simulink model "ssc_lithium_cell_1RC_testPulseData"  (R2022b)
settings: Solver=ode15s  StartTime=0.0  StopTime=40000  MaxStep=60  RelTol=1e-3  EnableMultiTasking=on
PreLoadFcn:
  | ssc_lithium_cell_1RC_ini
undefined symbols (not defined in the file or in its folder): sigbuilder_block
libraries: fl_lib x6, nesl_utility x4, LiBatteryBlocks x1
Description:
  | Lithium Battery Cell - One RC-Branch Equivalent Circuit
  | 
  | This example shows how to model a lithium cell using the Simscape(TM)
  | language to implement the elements of an equivalent circuit model
  | with one RC branch. For the defining equations and their validation,
  | see T. Huria, M. Ceraolo, J. Gazzarri, R. Jackey. "High Fidelity Electrical
  | Model with Thermal Dependence for Characterization and Simulation of
  | High Power Lithium Battery Cells," IEEE International Electric Vehicle
  | Conference, March 2012.
  | 
  | A simple thermal model is used to model battery temperature. It is
  | assumed that cooling is primarily via convection, and that heating is
  | primarily from internal resistance. A battery pack can be modeled by
  | connecting multiple copies of the battery cell block in series.
  | 
  | 
  | 
  | Copyright 2008-2012 The MathWorks, Inc.
settings Model: Creator=MathWorks  LastModifiedBy=Loki
settings SolverCC: AlgebraicLoopSolver=TrustRegion
settings DataIOCC: ExternalInput=[PulseData.time, PulseData.current, PulseData.temperature]  LimitDataPoints=on  LoadExternalInput=on  SaveFormat=Array  SignalLoggingSaveFormat=ModelDataLogs  ReturnWorkspaceOutputs=off
settings OptimizationCC: ExpressionDepthLimit=2147483647  LifeSpan=inf
settings DebuggingCC: UnderspecifiedInitializationDetection=Classic  MergeDetectMultiDrivingBlocksExec=none  FcnCallInpInsideContextMsg=warning  UnconnectedInputMsg=warning  UnconnectedOutputMsg=warning  UnconnectedLineMsg=warning  StateNameClashWarn=warning  SFUnexpectedBacktrackingDiag=warning  SFNoUnconditionalDefaultTransitionDiag=warning  SFExecutionAtInitializationDiag=none  SFMachineParentedDataDiag=warning  ArithmeticOperatorsInVariantConditions=warning
settings HardwareCC: ProdBitPerPointer=32  ProdBitPerSizeT=32  ProdBitPerPtrDiffT=32  ProdLargestAtomicFloat=None  ProdIntDivRoundTo=Undefined  ProdEndianess=Unspecified  ProdWordSize=32  ProdHWDeviceType=32-bit Generic
settings ModelReferenceCC: EnableRefExpFcnMdlSchedulingChecks=on  PropagateSignalLabelsOutOfModel=off
settings SFSimCC: SimUseLocalCustomCode=off  CustomCodeUndefinedFunction=UseInterfaceOnly
settings RTWCC: RTWUseLocalCustomCode=off
settings CodeAppCC: StateflowObjectComments=on
settings GRTTargetCC: TargetLangStandard=C89/C90 (ANSI)  CombineOutputUpdateFcns=off  GRTInterface=on
settings ConfigComp: CovMetricSettings=dw  CovSaveCumulativeToWorkspaceVar=on  CovSaveSingleToWorkspaceVar=on  CovExternalEMLEnable=off
settings SimscapeCC: SimscapeNormalizeSystem=off

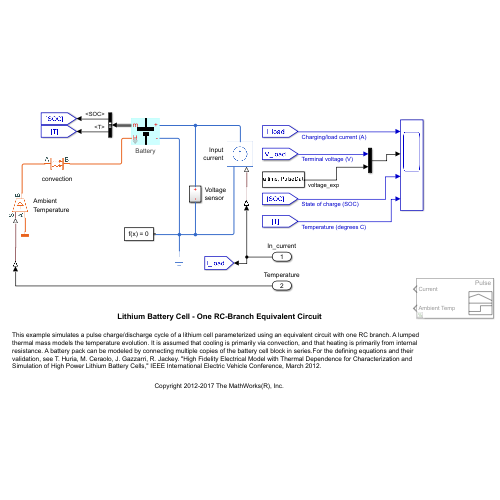
[thumbnail: Simulink's stored preview of the top-level diagram]
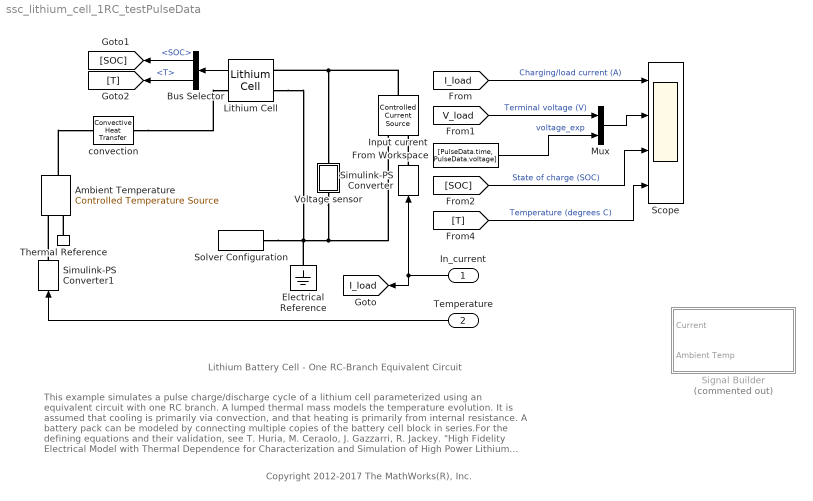
== system ssc_lithium_cell_1RC_testPulseData ==
  note: Lithium Battery Cell - One RC-Branch Equivalent Circuit
  note: This example simulates a pulse charge/discharge cycle of a lithium cell parameterized using an equivalent circuit with one RC branch. A lumped thermal mass models the temperature evolution. It is assumed that cooling is primarily via convection, and that heating is primarily from internal resistance. A battery pack can be modeled by connecting multiple copies of the battery cell block in series.For the defining equations and their validation, see T. Huria, M. Ceraolo, J. Gazzarri, R. Jackey. "High Fidelity Electrical Model with Thermal Dependence for Characterization and Simulation of High Power Lithium Battery Cells," IEEE International Electric Vehicle Conference, March 2012.
  note: Copyright 2012-2017 The MathWorks(R), Inc.
  In_current : Inport
  Temperature : Inport  Port=2
  Ambient Temperature : fl_lib/Thermal/Thermal Sources/Controlled Temperature Source
  Bus Selector : BusSelector  OutputSignals=SOC,T
  Electrical Reference : fl_lib/Electrical/Electrical Elements/Electrical Reference
  From Workspace : FromWorkspace  VariableName=[PulseData.time, PulseData.voltage]
  Input current : fl_lib/Electrical/Electrical Sources/Controlled Current Source
  Lithium Cell : LiBatteryBlocks/Lithium Cell  Battery=Battery
      settings: AttributesFormatString=%<Battery>
  Mux : Mux  Inputs=2
  Scope : Scope  NumInputPorts=4
  Signal Builder : Subsystem  Tag=STV Subsys  Commented=on  LoadFcn=sigbuilder_block('load');  StartFcn=sigbuilder_block('start');  StopFcn=sigbuilder_block('stop');  ClipboardFcn=sigbuilder_block('clipboard');  mask(Sigbuilder block){tuvar=[0:10]}
      mask help: Simulink:masks:SigbuilderBlock_MD
      mask init:
      | if ~strcmp(get_param(bdroot(gcbh),'SimulationStatus'),'stopped') tuvar = sigbuilder_block('maskInit'); end
      settings: CopyFcn=sigbuilder_block('copy');  DeleteFcn=sigbuilder_block('delete');  ModelCloseFcn=sigbuilder_block('modelClose');  PreSaveFcn=sigbuilder_block('preSave');  PauseFcn=sigbuilder_block('pause');  ContinueFcn=sigbuilder_block('continue');  NameChangeFcn=sigbuilder_block('namechange');  OpenFcn=sigbuilder_block('open',[33.75 101.25 755.25 399.75 ]);  CloseFcn=sigbuilder_block('close');
      mask Display: plot(0, 0, 100, 100,[2, 2, 32, 32, 2], [68, 8, 8, 68, 68],[32, 2], [38, 38], [32, 19, 2],[53, 60, 44], [32, 17, 17, 2],[16, 16, 31, 31]);txt = getActiveGroup(gcbh);text(2, 100, txt,'verticalAlignment', 'top');
  Simulink-PS Converter : nesl_utility/Simulink-PS Converter  PhysicalDomain=network_engine_domain  SubClassName=ps_input  LeftPortType=input  RightPortType=output  PseudoPeriodic=off  Frequencies=[]  NoiseDistribution=none  NoiseParameters=[]  Unit=A  AffineConversion=off  FilteringAndDerivatives=zero  SimscapeFilterOrder=1  InputFilterTimeConstant=.001  UdotUserProvided=1
  Simulink-PS Converter1 : nesl_utility/Simulink-PS Converter  PhysicalDomain=network_engine_domain  SubClassName=ps_input  LeftPortType=input  RightPortType=output  PseudoPeriodic=off  Frequencies=[]  NoiseDistribution=none  NoiseParameters=[]  Unit=degC  AffineConversion=on  FilteringAndDerivatives=zero  SimscapeFilterOrder=1  InputFilterTimeConstant=.001  UdotUserProvided=1
  Solver Configuration : nesl_utility/Solver Configuration  PhysicalDomain=network_engine_domain  SubClassName=solver  LeftPortType=input  RightPortType=generic  Tones=[]  Harmonics=[]  SimulateNoise=off  Profile=off  UseLocalSampling=off  EnableSwitchedLinearOptims=on  FrequencyDomain=off  UseCCode=off  RelTol=0.001  AbsTol=1e-06  MinStep=1e-09  ToWorkspace=off  RevertToSquareIcSolve=off  NumHomotopyIterations=100  PhasorMode=off  PhasorModeNumHarmonics=1  ConsistencySolver=NEWTON_FTOL  IndexReductionMethod=DerivativeReplacement  DoDC=off  ResidualTolerance=1e-9  ConsistencyTolSource=GLOBAL  ConsistencyAbsTol=0.001  ConsistencyRelTol=0.001  ConsistencyTolFactor=0.001  UseLocalSolver=off  LocalSolverChoice=NE_BACKWARD_EULER_ADVANCER  ResolveIndetEquations=on  FunctionEvalNumThread=1  LocalSolverSampleTime=1  DoFixedCost=off  MaxNonlinIter=3  MaxModeIter=2  ComputeImpulses=off  ImpulseIterations=2  LinearAlgebra=Sparse  LinearAlgebraNumThread=0  EquationFormulation=NE_TIME_EF  DelaysMemoryBudget=1024  AutomaticFiltering=on  FilteringTimeConstant=0.001  PartitionStorageMethod=AS_NEEDED  PartitionMemoryBudget=1024  PartitionMethod=FAST
  Thermal Reference : fl_lib/Thermal/Thermal Elements/Thermal Reference
  Voltage sensor : Subsystem
  convection : fl_lib/Thermal/Thermal Elements/Convective Heat Transfer  thermal_type=foundation.enum.constant_variable.constant  area=cell_area m^2  heat_tr_coeff=h_conv W/(m^2 * K)  min_heat_tr_coeff=1e-3 W/(K*m^2)  T_specify=off  T_priority=None  T=0 K  T_nominal_specify=off  T_nominal_unit=K  T_nominal_value=1  Q_specify=off  Q_priority=None  Q=0 J/s  Q_nominal_specify=off  Q_nominal_unit=J/s  Q_nominal_value=1
  tag scope: I_load=global
  wires:
  [SOC] -> Scope/3  "State of charge (SOC)"
  [T] -> Scope/4  "Temperature (degrees C)"
  [I_load] -> Scope/1  "Charging/load current (A)"
  In_current/1 -> [I_load], Simulink-PS Converter/1
  Lithium Cell/1 -> Bus Selector/1
  Bus Selector/1 -> [SOC]  "<SOC>"
  Bus Selector/2 -> [T]  "<T>"
  [V_load] -> Mux/1  "Terminal voltage (V)"
  Mux/1 -> Scope/2
  From Workspace/1 -> Mux/2  "voltage_exp"
  Temperature/1 -> Simulink-PS Converter1/1
  connections:
  Electrical Reference/LConn1 -- Input current/RConn2 -- Voltage sensor/RConn1 -- Lithium Cell/LConn2 -- Solver Configuration/RConn1
  Input current/LConn1 -- Lithium Cell/LConn1 -- Voltage sensor/LConn1
  Thermal Reference/LConn1 -- Ambient Temperature/RConn2
  Ambient Temperature/LConn1 -- convection/LConn1
  convection/RConn1 -- Lithium Cell/RConn1
  Simulink-PS Converter/RConn1 -- Input current/RConn1
  Simulink-PS Converter1/RConn1 -- Ambient Temperature/RConn1

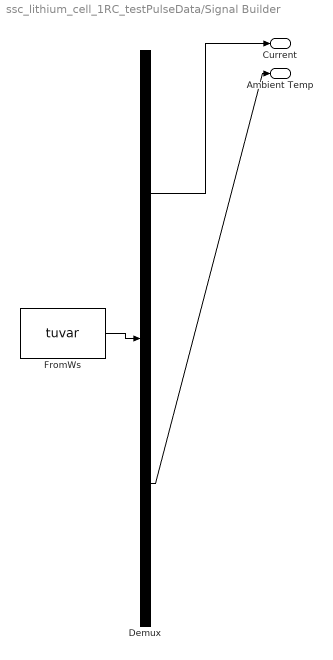
== system ssc_lithium_cell_1RC_testPulseData/Signal Builder ==
  Demux : Demux  Tag=STV Demux  Outputs=2
      settings: DisplayOption=none
  FromWs : FromWorkspace  Tag=STV FromWs  VariableName=tuvar
      SigBuilderData=|
      | common.afterFinalStr = 'Extrapolate'
      | common.sampleTime = 0
      | dataSet(1).timeRange = [0 40000]
      | dataSet(1).name = 'Pulse'
      | dataSet(2).timeRange = [0 40000]
      | dataSet(2).name = 'Constant'
      | sbobj.Name = 'Signal Builder'
      | sbobj.Groups(1).Name = 'Pulse'
      | sbobj.Groups(1).Signals(1).Name = 'Current'
      | sbobj.Groups(1).Signals(1).XData = [0 300 300 2100 2100 3600 3600 3960 3960 7200 7200 7560 7560 10800 10800 11160 11160 14400 14400 14760 14760 18000 18000 18360 18360 21600 21600 21960 21960 25200 25200 25560 25560 28800 28800 29160 29160 32400 32400 32760 32760 36000 36000 36360 36360 40000]
      | sbobj.Groups(1).Signals(1).YData = [0 0 31.5 31.5 0 0 -27.625 -27.625 0 0 -27.625 -27.625 0 0 -27.625 -27.625 0 0 -27.625 -27.625 0 0 -27.625 -27.625 0 0 -27.625 -27.625 0 0 -27.625 -27.625 0 0 -27.625 -27.625 0 0 -27.625 -27.625 0 0 -27.625 -27.625 0 0]
      | sbobj.Groups(1).Signals(2).Name = 'Ambient Temp'
      | sbobj.Groups(1).Signals(2).XData = [0 300 2100 3600 3960 7200 7560 10800 11160 14400 14760 18000 18360 21600 21960 25200 25560 28800 29160 32400 32760 36000 36360 40000]
      | sbobj.Groups(1).Signals(2).YData = [20 20 20 20 20 20 20 20 20 20 20 20 20 20 20 20 20 20 20 20 20 20 20 20]
      | sbobj.Groups(1).TimeRange = [0 40000]
      | sbobj.Groups(2).Name = 'Constant'
      | sbobj.Groups(2).Signals(1).Name = 'Current'
      | sbobj.Groups(2).Signals(1).XData = [0 360 360 9100 9100 11800 11800 28200 33800 40000]
      | sbobj.Groups(2).Signals(1).YData = [0 0 -5 -5 0 0 5 5 0 0]
      | sbobj.Groups(2).Signals(2).Name = 'Ambient Temp'
      | sbobj.Groups(2).Signals(2).XData = [0 360 360 9100 9100 11800 11800 28200 33800 40000]
      | sbobj.Groups(2).Signals(2).YData = [20 20.09 20.09 22.275 22.275 22.95 22.95 27.05 28.45 30]
      | sbobj.Groups(2).TimeRange = [0 40000]
  Current : Outport
  Ambient Temp : Outport  Tag=STV Outport  Port=2
  wires:
  Demux/1 -> Current/1
  FromWs/1 -> Demux/1
  Demux/2 -> Ambient Temp/1

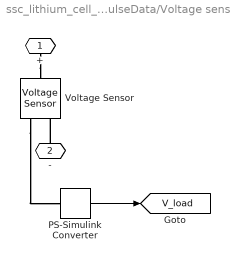
== system ssc_lithium_cell_1RC_testPulseData/Voltage sensor ==
  PS-Simulink Converter : nesl_utility/PS-Simulink Converter  PhysicalDomain=network_engine_domain  SubClassName=ps_output  LeftPortType=input  RightPortType=output  PseudoPeriodic=off  Frequencies=[]  VectorFormat=1-D array  Unit=V  AffineConversion=off
  Voltage Sensor : fl_lib/Electrical/Electrical Sensors/Voltage Sensor
  + : PMIOPort  Side=Left
  - : PMIOPort  Port=2  Side=Right
  tag scope: V_load=global
  wires:
  PS-Simulink Converter/1 -> [V_load]
  connections:
  Voltage Sensor/RConn1 -- PS-Simulink Converter/LConn1
  +/RConn1 -- Voltage Sensor/LConn1
  -/RConn1 -- Voltage Sensor/RConn2
